simulink model "Waehrungsmodelle"  (R2014a)
settings: Solver=ode1  StartTime=0.0  StopTime=100  FixedStep=1  MaxStep=1  MinStep=1  RelTol=1e-3
(part 8 of 18)

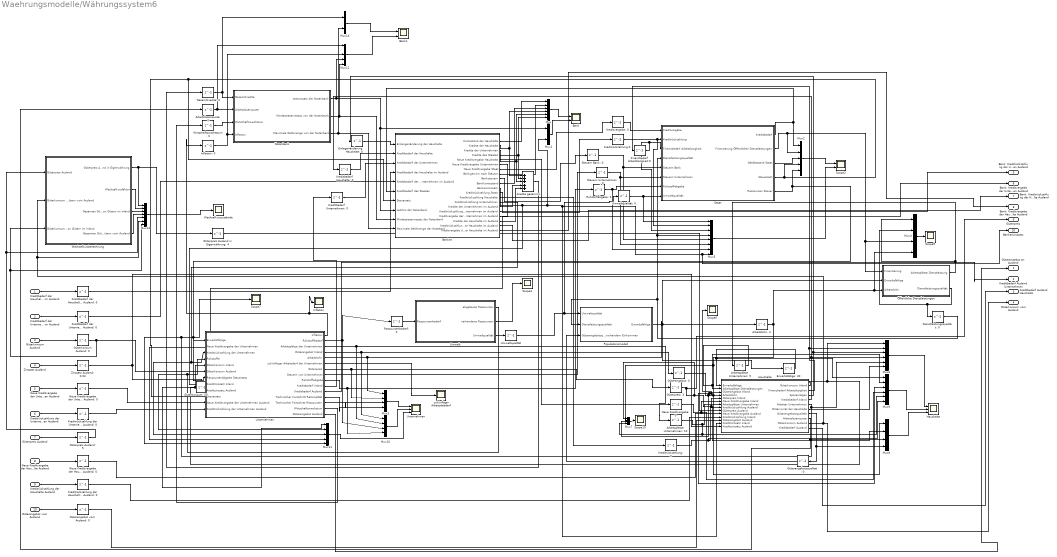
== system Waehrungsmodelle/Währungssystem6 ==
  Kreditbedarf der Haushalte im Ausland : Inport
  Kreditbedarf der Unternehmen im Ausland : Inport  Port=2
  Güterkonsum Ausland : Inport  Port=3
  Zinssatz Ausland : Inport  Port=4
  Neue Kreditvergabe der Unternehmen Ausland : Inport  Port=5
  Kreditrückzahlung der Unternehmen Ausland : Inport  Port=6
  Güterpreis Ausland : Inport  Port=7
  Neue Kreditvergabe der Haushalte Ausland : Inport  Port=8
  Kreditrückzahlung der Haushalte Ausland : Inport  Port=9
  Güterangebot vom  Ausland : Inport  Port=10
  Arbeitslohn: 4 : Delay  DelayLength=1  InitialCondition=4
  Arbeitslosenquote: 0 : Delay  DelayLength=1  InitialCondition=0
  "Arbeitsplätze Unternehmen: 10 " : Delay  DelayLength=1  InitialCondition=10
  Arbeitsplätze Unternehmen: 5 : Delay  DelayLength=1  InitialCondition=5
  Bank : Scope  NumInputPorts=2
      settings: ShowLegends=on  TimeRange=20  YMin=-500~0  YMax=500~0.1
  Bank1 : Scope  NumInputPorts=2
      settings: ShowLegends=on  TimeRange=20  YMin=-500~-0.5  YMax=10000~0.5  SaveName=ScopeData3
  Banken : Subsystem
  Dienstleistungsqualität: 0 : Delay  DelayLength=1  InitialCondition=0
  Einlagenänderung Haushalte: 0 : Delay  DelayLength=1  InitialCondition=0
  Erwerbstätige: 30 : Delay  DelayLength=1  InitialCondition=30
  Finanzbedarf Arbeitslosigkeit:0 : Delay  DelayLength=1  InitialCondition=0
  Gesamtkredite: 0 : Delay  DelayLength=1  InitialCondition=0
  Güterangebot vom  Ausland: 0 : Delay  DelayLength=1  InitialCondition=0
  Güterangebot: 0 : Delay  DelayLength=1  InitialCondition=0
  Güterangebotsqualität: 0 : Delay  DelayLength=1  InitialCondition=0
  Güterkonsum Ausland: 0 : Delay  DelayLength=1  InitialCondition=0
  Güterkonsum: 50 : Delay  DelayLength=1  InitialCondition=50
  Güterpreis Ausland in Eigenwährung: 4 : Delay  DelayLength=1  InitialCondition=4
  Güterpreis Ausland: 5 : Delay  DelayLength=1  InitialCondition=5
  Güterpreis: 3 : Delay  DelayLength=1  InitialCondition=3
  Haushalte : Subsystem
  "Haushalte " : Scope  NumInputPorts=3
      settings: TickLabels=on  ShowLegends=on  TimeRange=100  YMin=-50~0~0  YMax=150~100~1
  Inflation : Scope
      settings: ShowLegends=on  TimeRange=100  YMin=-0.1  YMax=0.15  SaveName=ScopeData12
  Inflation: 0 : Delay  DelayLength=1  InitialCondition=0
  Kreditbedarf Haushalte: 0 : Delay  DelayLength=1  InitialCondition=0
  Kreditbedarf Unternehmen: 0 : Delay  DelayLength=1  InitialCondition=0
  Kreditbedarf der Haushalte im Ausland: 0 : Delay  DelayLength=1  InitialCondition=0
  Kreditbedarf der Unternehmen im Ausland: 0 : Delay  DelayLength=1  InitialCondition=0
  Kredite gesammt : Sum  Inputs=+++++
  Kreditrückzahlung der Haushalte Ausland: 0 : Delay  DelayLength=1  InitialCondition=0
  Kreditrückzahlung der Unternehmen Ausland: 0 : Delay  DelayLength=1  InitialCondition=0
  Kreditrückzahlung: 0 : Delay  DelayLength=1  InitialCondition=0
  Kreditrückzahlung:0 : Delay  DelayLength=1  InitialCondition=0
  Kreditvergabe: 0 : Delay  DelayLength=1  InitialCondition=0
  Mux : Mux  Inputs=6
  Mux1 : Mux  Inputs=2
  Mux{3..4,7..8,10} (5 alike) : Mux
  Mux11 : Mux  Inputs=5
  Mux12 : Mux  Inputs=5
  Mux13 : Mux  Inputs=7
  Mux14 : Mux  Inputs=2
  Mux2 : Mux  Inputs=5
  Mux5 : Mux  Inputs=8
  Mux6 : Mux  Inputs=6
  Mux9 : Mux  Inputs=6
  Neue Kreditvergabe der Haushalte Ausland: 0 : Delay  DelayLength=1  InitialCondition=0
  Neue Kreditvergabe der Unternehmen Ausland: 0 : Delay  DelayLength=1  InitialCondition=0
  Neue Kreditvergabe: 0 : Delay  DelayLength=1  InitialCondition=0
  Notenbank : Subsystem
  Populationsmodell : Subsystem
  Ressourcenbedarf: 0 : Delay  DelayLength=1  InitialCondition=0
  Rohstoffabgabe: 0 : Delay  DelayLength=1  InitialCondition=0
  Scope{4..5,7,9..10} (5 alike) : Scope
      Scope10 settings: ShowLegends=on  TimeRange=100  YMin=0  YMax=120  SaveName=ScopeData10
      Scope4 settings: SaveName=ScopeData4
      Scope5 settings: TimeRange=10  YMin=0  YMax=10  SaveName=ScopeData5
      Scope7 settings: ShowLegends=on  TimeRange=10  YMin=9  YMax=15  SaveName=ScopeData7
      Scope9 settings: TickLabels=on  ShowLegends=on  TimeRange=100  YMin=0  YMax=40  SaveName=ScopeData9
  Scope2 : Scope  NumInputPorts=2
      settings: ShowLegends=on  TimeRange=100  YMin=-100~0  YMax=300~500  SaveName=ScopeData2
  Staat : Subsystem
  Steuern Bank: 0 : Delay  DelayLength=1  InitialCondition=0
  Steuern Unternehmen: 0 : Delay  DelayLength=1  InitialCondition=0
  Umwelt : Subsystem
  Umweltqualität : Delay  DelayLength=1  InitialCondition=0
  Umweltqualität: 0 : Delay  DelayLength=1  InitialCondition=0
  Unternehmen : Subsystem
  "Unternehmen " : Scope  NumInputPorts=3
      settings: TickLabels=on  ShowLegends=on  TimeRange=100  YMin=2~-5~-5  YMax=50~200~100  SaveName=ScopeData6
  Wechselkursberechnung : Subsystem
  Wechselkurszustände : Scope
      settings: ShowLegends=on  TimeRange=100  YMin=0  YMax=1  SaveName=ScopeData11
  Wirtschaftswachtstum: 0 : Delay  DelayLength=1  InitialCondition=0
  Zinssatz Ausland: 0.03 : Delay  DelayLength=1  InitialCondition=0.03
  zukünftiger Arbeitsdebdarf : Scope
      settings: ShowLegends=on  TimeRange=10  YMin=9  YMax=15  SaveName=ScopeData14
  Öffentliche Dienstleistungen : Subsystem
  Güterangebot an  Ausland : Outport
  Kreditbedarf Ausland Unternehmen : Outport  Port=2
  Kreditbedarf Ausland Haushalte : Outport  Port=3
  Güterkonsum vom Ausland : Outport  Port=4
  Bank: Kreditrückzahlung der Unternemen Ausland : Outport  Port=5
  "Bank: Kreditvergabe der Unternemen Ausland " : Outport  Port=6
  Bank: Kreditrückzahlung der Haushalte Ausland : Outport  Port=7
  "Bank: Kreditvergabe der Haushalte Ausland " : Outport  Port=8
  Güterpreis : Outport  Port=9
  Bankenzinssatz : Outport  Port=10
  wires:
  Öffentliche Dienstleistungen/1(Arbeitsplätze Dienstleistung) -> Arbeitsplätze Unternehmen: 5/1, Mux4/1
  Staat/4(Steuersatz) -> Mux2/4, Banken/7(Steuersatz), Unternehmen/10(Steuersatz)
  Umwelt/3(Umweltqualität) -> Umweltqualität/1
  Staat/5(Ressourcen Steuer) -> Unternehmen/7(RessourcenAbgabe Steuersatz), Mux2/5
  Populationsmodell/1(Erwerbsfähige) -> Erwerbstätige: 30/1, Öffentliche Dienstleistungen/2(Erwerbsfähige)
  Unternehmen/7(Güterpreis) -> Mux3/2, Güterpreis: 3/1
  Unternehmen/5(Arbeitslohn) -> Mux3/1, Arbeitslohn: 4/1
  Unternehmen/4(Güterangebot Inland) -> Mux10/1, Güterangebot: 0/1
  Unternehmen/3(Arbeitsplätze der Unternehmen) -> Mux10/2, "Arbeitsplätze Unternehmen: 10 "/1
  Umwelt/1(abgebaute Ressourcen) -> Unternehmen/4(Rohstoffe), Mux11/2
  Haushalte/1(Güterkonsum Inland) -> Mux6/1, Güterkonsum: 50/1
  Haushalte/7(Güterangebotsqualität) -> Mux8/4, Güterangebotsqualität: 0/1
  Staat/2(Finanzierung Öffentlicher Dienstleistungen) -> Mux2/2, Öffentliche Dienstleistungen/1(Finanzierung), Mux4/3
  Haushalte/5(Arbeiter Unternehmen) -> Mux6/5, Scope7/1, Unternehmen/1(Erwerbsfähige), Mux11/5
  Haushalte/2(Finanzbedarf Arbeitslosigkeit) -> Finanzbedarf Arbeitslosigkeit:0/1, Mux6/2
  Unternehmen/8(Steuern von Unternehmen) -> Steuern Unternehmen: 0/1
  Unternehmen/9(Rohstoffabgabe) -> Mux10/4, Rohstoffabgabe: 0/1
  Haushalte/8(Arbeitslosenquote) -> Arbeitslosenquote: 0/1, Mux8/3
  Unternehmen/1(Inflation) -> Inflation/1, Inflation: 0/1
  Unternehmen/14(Wirtschaftswachstum) -> Wirtschaftswachtstum: 0/1
  Notenbank/1(Leitzinssatz der Notenbank) -> Mux12/4, Mux1/1, Banken/8(Leitzins der Notenbank)
  Notenbank/2(Mindestreservesatz von der Notenbank) -> Mux12/5, Banken/9(Mindestreservesatz der Notenbank)
  Notenbank/3(Maximale Geldmenge von der Notenbank) -> Banken/10(Maximale Geldmenge der Notebank), Mux14/2
  Banken/2(Kredite der Haushalte) -> Mux/4, Kredite gesammt/1
  Banken/3(Kredite der Unternehmen) -> Mux/6, Kredite gesammt/2
  Banken/4(Kredite des Staates) -> Mux/5, Kredite gesammt/3
  Banken/9(Banksteuern) -> Steuern Bank: 0/1
  Banken/7(Neue Kreditvergabe Staat) -> Kreditvergabe: 0/1
  Banken/12(Kreditrückzahlung Staat) -> Kreditrückzahlung:0/1
  Banken/13(Kreditrückzahlung Haushalte) -> Kreditrückzahlung: 0/1
  Banken/5(Neue Kreditvergabe Haushalte) -> Neue Kreditvergabe: 0/1
  Haushalte/3(Spareinlagen) -> Einlagenänderung Haushalte: 0/1, Mux6/3
  Haushalte/4(Kreditbedarf Inland) -> Kreditbedarf Haushalte: 0/1, Mux6/4
  Unternehmen/10(Kreditbedarf Inland) -> Kreditbedarf Unternehmen: 0/1
  Staat/1(Kreditbedarf) -> Banken/6(Kreditbedarf des Staates), Mux2/1
  Banken/6(Neue Kreditvergabe Unternehmen) -> Mux11/4, Unternehmen/2(Neue Kreditvergabe der Unternehmen)
  Banken/14(Kreditrückzahlung Unternehmen) -> Unternehmen/3(Kreditrückzahlung der Unternehmen), Mux11/3
  Banken/1(Kontostand der Haushalte) -> Mux/1
  Banken/8(Bankgewinn nach Steuern) -> Mux/2
  Banken/10(Bankkontostand) -> Mux/3
  Banken/11(Bankenzinssatz) -> Haushalte/13(Kreditzinssatz Inland), Bankenzinssatz/1, Mux5/8, Mux1/2, Unternehmen/8(Kreditzinssatz Inland)
  Unternehmen/13(Technischer Fortschritt Ressourcen) -> Mux3/3
  Unternehmen/12(Technischer Fortschritt Rationalität) -> Mux3/4
  Umwelt/2(verhandene Ressourcen) -> Scope4/1
  Kredite gesammt/1 -> Gesamtkredite: 0/1
  Gesamtkredite: 0/1 -> Notenbank/1(Gesamtkredite), Mux14/1
  Wirtschaftswachtstum: 0/1 -> Notenbank/3(Wirtschaftswachtsum)
  Inflation: 0/1 -> Mux12/3, Notenbank/4(Inflation)
  Ressourcenbedarf: 0/1 -> Umwelt/1(Ressourcenbedarf)
  Unternehmen/2(Rohstoffbedarf) -> Ressourcenbedarf: 0/1, Mux10/3
  Umweltqualität: 0/1 -> Mux5/1, Staat/8(Umweltqualität)
  Rohstoffabgabe: 0/1 -> Mux5/7, Staat/7(Rohstoffabgabe)
  Dienstleistungsqualität: 0/1 -> Populationsmodell/2(Dienstleistungsqualität), Staat/4(Dienstleistungsqualität), Mux5/4
  Steuern Unternehmen: 0/1 -> Mux5/6, Staat/6(Steuern Unternehmen)
  Steuern Bank: 0/1 -> Staat/5(Steuern Bank), Mux5/5
  Finanzbedarf Arbeitslosigkeit:0/1 -> Mux5/3, Staat/3(Finanzbedarf Arbeitslosigkeit)
  Kreditrückzahlung:0/1 -> Staat/2(Kreditrückzahlung), Mux5/2
  Kreditvergabe: 0/1 -> Staat/1(Kreditvergabe)
  Umweltqualität/1 -> Umweltqualität: 0/1, Populationsmodell/1(Umweltqualität)
  Öffentliche Dienstleistungen/2(Dienstleistungsqualität) -> Dienstleistungsqualität: 0/1, Mux4/2
  Güterangebotsqualität: 0/1 -> Populationsmodell/3(Güterangebotsqualität bei vorhandem Einkommen)
  "Arbeitsplätze Unternehmen: 10 "/1 -> Mux9/5, Mux7/4, Haushalte/7(Arbeitsplätze Unternehmen)
  Kreditrückzahlung: 0/1 -> Mux9/6, Haushalte/8(Kreditrückzahlung Ausland)
  Neue Kreditvergabe: 0/1 -> Mux9/4, Haushalte/6(Neue Kreditvergabe Inland)
  Arbeitslohn: 4/1 -> Mux8/1, Haushalte/4(Arbeitslohn), Mux7/2, Mux4/4, Öffentliche Dienstleistungen/3(Arbeitslohn)
  Güterangebot: 0/1 -> Mux7/3, Mux9/3, Haushalte/3(Güterangebot Inland), Scope5/1
  Arbeitsplätze Unternehmen: 5/1 -> Haushalte/2(Arbeitsplätze Dienstleistungen), Mux9/2
  Erwerbstätige: 30/1 -> Haushalte/1(Erwerbsfähige), Mux9/1
  Güterkonsum: 50/1 -> Unternehmen/5(Güterkonsum Inland), Mux11/1
  Mux4/1 -> Scope9/1
  Staat/3(Geldbestand Staat) -> Mux2/3
  Mux2/1 -> Scope2/1
  Mux5/1 -> Scope2/2
  Mux/1 -> Bank/1
  Mux7/1 -> Scope10/1
  Mux1/1 -> Bank/2
  Mux6/1 -> "Haushalte "/1
  Mux8/1 -> "Haushalte "/3
  Haushalte/6(Gütervorrat der Haushalte) -> Mux6/6
  Mux9/1 -> "Haushalte "/2
  Mux3/1 -> "Unternehmen "/1
  Mux10/1 -> "Unternehmen "/2
  Mux11/1 -> "Unternehmen "/3
  Güterkonsum Ausland/1 -> Güterkonsum Ausland: 0/1
  Zinssatz Ausland: 0.03/1 -> Haushalte/14(Kreditzinssatz Ausland), Unternehmen/9(Kreditzinssatz Ausland)
  Unternehmen/15(Güterangebot Ausland) -> Güterangebot an  Ausland/1
  Kreditbedarf Haushalte: 0/1 -> Banken/2(Kreditbedarf der Haushalte)
  Kreditbedarf Unternehmen: 0/1 -> Banken/3(Kreditbedarf der Unternehmen)
  Einlagenänderung Haushalte: 0/1 -> Banken/1(Einlangenänderung der Haushalte)
  Kreditbedarf der Haushalte im Ausland: 0/1 -> Banken/4(Kreditbedarf der Haushalte im Ausland)
  Kreditbedarf der Unternehmen im Ausland: 0/1 -> Banken/5(Kreditbedarf der Unternehmen im Ausland)
  Neue Kreditvergabe der Unternehmen Ausland/1 -> Neue Kreditvergabe der Unternehmen Ausland: 0/1
  Kreditrückzahlung der Unternehmen Ausland/1 -> Kreditrückzahlung der Unternehmen Ausland: 0/1
  Banken/16(Kreditrückzahlung der Unternehmen im Ausland) -> Bank: Kreditrückzahlung der Unternemen Ausland/1
  Banken/18(Kredite der Haushalte im Ausland) -> Kredite gesammt/5
  Banken/15(Kredite der Unternehmen im Ausland) -> Kredite gesammt/4
  Neue Kreditvergabe der Haushalte Ausland/1 -> Neue Kreditvergabe der Haushalte Ausland: 0/1
  Unternehmen/11(Kreditbedarf Ausland) -> Kreditbedarf Ausland Unternehmen/1
  Kreditrückzahlung der Haushalte Ausland/1 -> Kreditrückzahlung der Haushalte Ausland: 0/1
  Haushalte/10(Kreditbedarf Ausland) -> Kreditbedarf Ausland Haushalte/1
  Banken/20(Kreditvergabe der Haushalte im Ausland) -> "Bank: Kreditvergabe der Haushalte Ausland "/1
  Güterangebot vom  Ausland/1 -> Güterangebot vom  Ausland: 0/1
  Unternehmen/6(zukünftiger Arbeitsdarf der Unternehmen) -> zukünftiger Arbeitsdebdarf/1
  Banken/17(Kreditvergabe der Unternehmen im Ausland) -> "Bank: Kreditvergabe der Unternemen Ausland "/1
  Banken/19(Kreditrückzahlung der Haushalte im Ausland) -> Bank: Kreditrückzahlung der Haushalte Ausland/1
  Güterpreis: 3/1 -> Güterpreis/1, Mux7/1, Mux8/2, Haushalte/5(Güterpreis Inland)
  Kreditbedarf der Haushalte im Ausland/1 -> Kreditbedarf der Haushalte im Ausland: 0/1
  Kreditbedarf der Unternehmen im Ausland/1 -> Kreditbedarf der Unternehmen im Ausland: 0/1
  Güterkonsum Ausland: 0/1 -> Mux13/7, Wechselkursberechnung/3(Güterkonsum im Ausland von Gütern im Inland), Unternehmen/6(Güterkonsum Ausland)
  Zinssatz Ausland/1 -> Zinssatz Ausland: 0.03/1
  Neue Kreditvergabe der Unternehmen Ausland: 0/1 -> Unternehmen/11(Neue Kreditvergabe der Unternehmen Ausland)
  Kreditrückzahlung der Unternehmen Ausland: 0/1 -> Unternehmen/12(Kreditrückzahlung der Unternehmen Ausland)
  Güterpreis Ausland: 5/1 -> Mux13/5, Wechselkursberechnung/1(Güterpreis Ausland)
  Neue Kreditvergabe der Haushalte Ausland: 0/1 -> Haushalte/10(Neue Kreditvergabe Ausland)
  Kreditrückzahlung der Haushalte Ausland: 0/1 -> Haushalte/11(Kreditrückzahlung Inland)
  Güterangebot vom  Ausland: 0/1 -> Haushalte/12(Güterangebot Ausland)
  Mux14/1 -> Bank1/1
  Mux12/1 -> Bank1/2
  Arbeitslosenquote: 0/1 -> Notenbank/2(Arbeitslosenquote), Mux12/1
  Güterpreis Ausland/1 -> Güterpreis Ausland: 5/1
  Wechselkursberechnung/1(Güterpreis Ausland in Eigenwährung) -> Güterpreis Ausland in Eigenwährung: 4/1, Mux13/1
  Haushalte/9(Güterkonsum Ausland) -> Mux13/6, Wechselkursberechnung/2(Güterkonsum im Inland von Gütern vom Ausland), Güterkonsum vom Ausland/1
  Güterpreis Ausland in Eigenwährung: 4/1 -> Haushalte/9(Güterpreis Ausland)
  Wechselkursberechnung/3(Gesamter Güterkonsum im Ausland von Gütern im Inland) -> Mux13/3
  Wechselkursberechnung/2(Wechselkursfaktor) -> Mux13/2
  Wechselkursberechnung/4(Gesamter Güterkonsum im Inland von Gütern vom Ausland) -> Mux13/4
  Mux13/1 -> Wechselkurszustände/1

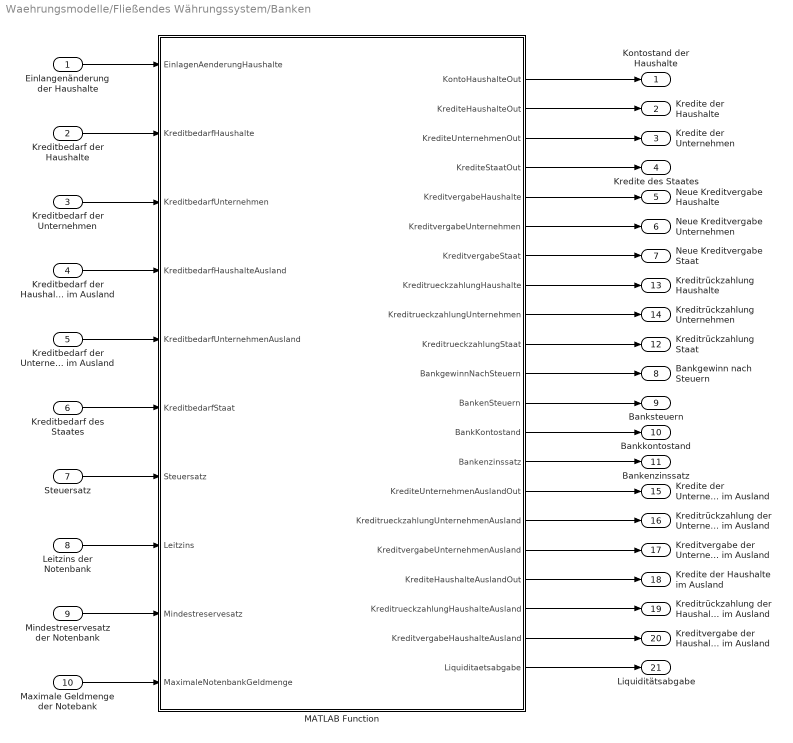
== system Waehrungsmodelle/Fließendes Währungssystem/Banken ==
  Einlangenänderung der Haushalte : Inport
  Kreditbedarf der Haushalte : Inport  Port=2
  Kreditbedarf der Unternehmen : Inport  Port=3
  Kreditbedarf der Haushalte im Ausland : Inport  Port=4
  Kreditbedarf der Unternehmen im Ausland : Inport  Port=5
  Kreditbedarf des Staates : Inport  Port=6
  Steuersatz : Inport  Port=7
  Leitzins der Notenbank : Inport  Port=8
  Mindestreservesatz der Notenbank : Inport  Port=9
  Maximale Geldmenge der Notebank : Inport  Port=10
  MATLAB Function : MATLAB Function  TreatAsAtomicUnit=on
  Kontostand der Haushalte : Outport
  Kredite der Haushalte : Outport  Port=2
  Kredite der Unternehmen : Outport  Port=3
  Kredite des Staates : Outport  Port=4
  Neue Kreditvergabe Haushalte : Outport  Port=5
  Neue Kreditvergabe Unternehmen : Outport  Port=6
  Neue Kreditvergabe Staat : Outport  Port=7
  Bankgewinn nach Steuern : Outport  Port=8
  Banksteuern : Outport  Port=9
  Bankkontostand : Outport  Port=10
  Bankenzinssatz : Outport  Port=11
  Kreditrückzahlung Staat : Outport  Port=12
  Kreditrückzahlung Haushalte : Outport  Port=13
  Kreditrückzahlung Unternehmen : Outport  Port=14
  Kredite der Unternehmen im Ausland : Outport  Port=15
  Kreditrückzahlung der Unternehmen im Ausland : Outport  Port=16
  Kreditvergabe der Unternehmen im Ausland : Outport  Port=17
  Kredite der Haushalte im Ausland : Outport  Port=18
  Kreditrückzahlung der Haushalte im Ausland : Outport  Port=19
  Kreditvergabe der Haushalte im Ausland : Outport  Port=20
  Liquiditätsabgabe : Outport  Port=21
  wires:
  MATLAB Function/1(KontoHaushalteOut) -> Kontostand der Haushalte/1
  MATLAB Function/2(KrediteHaushalteOut) -> Kredite der Haushalte/1
  MATLAB Function/3(KrediteUnternehmenOut) -> Kredite der Unternehmen/1
  MATLAB Function/4(KrediteStaatOut) -> Kredite des Staates/1
  MATLAB Function/5(KreditvergabeHaushalte) -> Neue Kreditvergabe Haushalte/1
  MATLAB Function/6(KreditvergabeUnternehmen) -> Neue Kreditvergabe Unternehmen/1
  MATLAB Function/7(KreditvergabeStaat) -> Neue Kreditvergabe Staat/1
  MATLAB Function/11(BankgewinnNachSteuern) -> Bankgewinn nach Steuern/1
  MATLAB Function/10(KreditrueckzahlungStaat) -> Kreditrückzahlung Staat/1
  MATLAB Function/9(KreditrueckzahlungUnternehmen) -> Kreditrückzahlung Unternehmen/1
  MATLAB Function/8(KreditrueckzahlungHaushalte) -> Kreditrückzahlung Haushalte/1
  MATLAB Function/14(Bankenzinssatz) -> Bankenzinssatz/1
  MATLAB Function/13(BankKontostand) -> Bankkontostand/1
  MATLAB Function/12(BankenSteuern) -> Banksteuern/1
  MATLAB Function/15(KrediteUnternehmenAuslandOut) -> Kredite der Unternehmen im Ausland/1
  MATLAB Function/16(KreditrueckzahlungUnternehmenAusland) -> Kreditrückzahlung der Unternehmen im Ausland/1
  MATLAB Function/17(KreditvergabeUnternehmenAusland) -> Kreditvergabe der Unternehmen im Ausland/1
  MATLAB Function/18(KrediteHaushalteAuslandOut) -> Kredite der Haushalte im Ausland/1
  MATLAB Function/20(KreditvergabeHaushalteAusland) -> Kreditvergabe der Haushalte im Ausland/1
  MATLAB Function/19(KreditrueckzahlungHaushalteAusland) -> Kreditrückzahlung der Haushalte im Ausland/1
  Einlangenänderung der Haushalte/1 -> MATLAB Function/1(EinlagenAenderungHaushalte)
  Kreditbedarf der Haushalte/1 -> MATLAB Function/2(KreditbedarfHaushalte)
  Kreditbedarf der Unternehmen/1 -> MATLAB Function/3(KreditbedarfUnternehmen)
  Kreditbedarf der Haushalte im Ausland/1 -> MATLAB Function/4(KreditbedarfHaushalteAusland)
  Kreditbedarf der Unternehmen im Ausland/1 -> MATLAB Function/5(KreditbedarfUnternehmenAusland)
  Kreditbedarf des Staates/1 -> MATLAB Function/6(KreditbedarfStaat)
  Steuersatz/1 -> MATLAB Function/7(Steuersatz)
  Leitzins der Notenbank/1 -> MATLAB Function/8(Leitzins)
  Mindestreservesatz der Notenbank/1 -> MATLAB Function/9(Mindestreservesatz)
  Maximale Geldmenge der Notebank/1 -> MATLAB Function/10(MaximaleNotenbankGeldmenge)
  MATLAB Function/21(Liquiditaetsabgabe) -> Liquiditätsabgabe/1

== system Waehrungsmodelle/Fließendes Währungssystem/Haushalte ==
  Erwerbsfähige : Inport
  Arbeitsplätze Dienstleistungen : Inport  Port=2
  Güterangebot Inland : Inport  Port=3
  Arbeitslohn : Inport  Port=4
  Güterpreis Inland : Inport  Port=5
  Neue Kreditvergabe Inland : Inport  Port=6
  Arbeitsplätze Unternehmen : Inport  Port=7
  Kreditrückzahlung Ausland : Inport  Port=8
  Güterpreis Ausland : Inport  Port=9
  Neue Kreditvergabe Ausland : Inport  Port=10
  Kreditrückzahlung Inland : Inport  Port=11
  Güterangebot Ausland : Inport  Port=12
  Kreditzinssatz Inland : Inport  Port=13
  Kreditzinssatz Ausland : Inport  Port=14
  MATLAB Function : MATLAB Function  TreatAsAtomicUnit=on
  Güterkonsum Inland : Outport
  Finanzbedarf Arbeitslosigkeit : Outport  Port=2
  Spareinlagen : Outport  Port=3
  Kreditbedarf Inland : Outport  Port=4
  Arbeiter Unternehmen : Outport  Port=5
  Gütervorrat der Haushalte : Outport  Port=6
  Güterangebotsqualität : Outport  Port=7
  Arbeitslosenquote : Outport  Port=8
  Güterkonsum Ausland : Outport  Port=9
  Kreditbedarf Ausland : Outport  Port=10
  wires:
  Arbeitslohn/1 -> MATLAB Function/7(Arbeitslohn)
  Erwerbsfähige/1 -> MATLAB Function/1(Erwerbsfaehige)
  Arbeitsplätze Dienstleistungen/1 -> MATLAB Function/2(ArbeitsplaetzeDienstleistungen)
  Güterangebot Inland/1 -> MATLAB Function/6(GueterAngebotInland)
  Güterpreis Inland/1 -> MATLAB Function/8(GueterpreisInland)
  MATLAB Function/1(GueterkonsumInland) -> Güterkonsum Inland/1
  MATLAB Function/2(FinanzierungArbeitslosigkeit) -> Finanzbedarf Arbeitslosigkeit/1
  MATLAB Function/4(KreditbedarfInland) -> Kreditbedarf Inland/1
  MATLAB Function/5(ArbeiterUnternehmen) -> Arbeiter Unternehmen/1
  MATLAB Function/3(Spareinlagen) -> Spareinlagen/1
  Neue Kreditvergabe Inland/1 -> MATLAB Function/4(NeueKreditvergabeInland)
  Arbeitsplätze Unternehmen/1 -> MATLAB Function/3(ArbeitsplaetzeUnternehmen)
  MATLAB Function/6(GueterVorratHaushalte) -> Gütervorrat der Haushalte/1
  MATLAB Function/7(GueterangebotsqualitaetOut) -> Güterangebotsqualität/1
  Kreditrückzahlung Ausland/1 -> MATLAB Function/5(KreditrueckzahlungInland)
  MATLAB Function/8(Arbeitslosenquote) -> Arbeitslosenquote/1
  MATLAB Function/9(GueterkonsumAusland) -> Güterkonsum Ausland/1
  MATLAB Function/10(KreditbedarfAusland) -> Kreditbedarf Ausland/1
  Güterpreis Ausland/1 -> MATLAB Function/9(GueterpreisAusland)
  Neue Kreditvergabe Ausland/1 -> MATLAB Function/10(NeueKreditvergabeAusland)
  Kreditrückzahlung Inland/1 -> MATLAB Function/11(KreditrueckzahlungAusland)
  Güterangebot Ausland/1 -> MATLAB Function/12(GueterAngebotAusland)
  Kreditzinssatz Inland/1 -> MATLAB Function/13(KreditZinssatzInland)
  Kreditzinssatz Ausland/1 -> MATLAB Function/14(KreditZinssatzAusland)

== system Waehrungsmodelle/Fließendes Währungssystem/Notenbank ==
  Gesamtkredite : Inport
  Arbeitslosenquote : Inport  Port=2
  Wirtschaftswachtsum : Inport  Port=3
  Inflation : Inport  Port=4
  MATLAB Function : MATLAB Function  TreatAsAtomicUnit=on
  Leitzinssatz der Notenbank : Outport
  Mindestreservesatz von der Notenbank : Outport  Port=2
  Maximale Geldmenge von der Notenbank : Outport  Port=3
  wires:
  MATLAB Function/2(MindestreservesatzOut) -> Mindestreservesatz von der Notenbank/1
  MATLAB Function/3(MaximaleNotenbankGeldmengeOut) -> Maximale Geldmenge von der Notenbank/1
  MATLAB Function/1(LeitzinsOut) -> Leitzinssatz der Notenbank/1
  Wirtschaftswachtsum/1 -> MATLAB Function/4(Wirtschaftswachtsum)
  Arbeitslosenquote/1 -> MATLAB Function/2(Arbeitslosenquote)
  Gesamtkredite/1 -> MATLAB Function/1(Gesamtkredite)
  Inflation/1 -> MATLAB Function/3(Inflation)

== system Waehrungsmodelle/Fließendes Währungssystem/Populationsmodell ==
  note: Geburten
  Umweltqualität : Inport
  Dienstleistungsqualität : Inport  Port=2
  Güterangebotsqualität bei vorhandem Einkommen : Inport  Port=3
  Ausgleichsfaktor : Constant  Value=0.3
  Dienstleistungs- multiplikator : Sum
  Divide1 : Product  Inputs=*/
  Divide2 : Product  Inputs=*/
  Divide3 : Product  Inputs=*/
  Erwachsene : Sum  Inputs=+--
  Fertilitätsmultiplikator : Product  Inputs=4
  Fertilitätsrate pro Frau : Constant  Value=3/40
  Frauenanteil pro Erwachsene : Constant  Value=0.5
  Güterangebotsqualitäts- multiplikator : Sum
  Jahre der Altersklasse : Constant  Value=15
  Jahre der Altersklasse1 : Constant  Value=10
  Jahre der Altersklasse2 : Constant  Value=40
  Kinder : Sum  Inputs=+--
  Lebensqualitätsfaktor : Product  Inputs=/
  Product{,1..3} (4 alike) : Product  Inputs=3
  Schüler / Studenten : Sum  Inputs=+--
  Start Erwachsene: 55 : Integrator  InitialCondition=55
  Start Kinder: 13 : Integrator  InitialCondition=13
  Start Schüler: 11 : Integrator  InitialCondition=11
  Sterblichkeitsrate Kinder : Constant  Value=0.003
  Sterblichkeitsrate1 : Constant  Value=0.002
  Sterblichkeitsrate2 : Constant  Value=0.004
  Umwelt- multiplikator : Sum
  Erwerbsfähige : Outport
  wires:
  Product/1 -> Kinder/1
  Jahre der Altersklasse2/1 -> Divide3/2
  Jahre der Altersklasse/1 -> Divide1/2
  Divide1/1 -> Schüler / Studenten/1, Kinder/3
  Sterblichkeitsrate1/1 -> Product1/2
  Sterblichkeitsrate Kinder/1 -> Product2/2
  Divide2/1 -> Schüler / Studenten/3, Erwachsene/1
  Start Schüler: 11/1 -> Product1/3, Divide2/1
  Jahre der Altersklasse1/1 -> Divide2/2
  Sterblichkeitsrate2/1 -> Product3/2
  Start Erwachsene: 55/1 -> Erwerbsfähige/1, Product3/3, Divide3/1, Product/1
  Erwachsene/1 -> Start Erwachsene: 55/1
  Kinder/1 -> Start Kinder: 13/1
  Start Kinder: 13/1 -> Product2/3, Divide1/1
  Schüler / Studenten/1 -> Start Schüler: 11/1
  Ausgleichsfaktor/1 -> Umwelt- multiplikator/2, Güterangebotsqualitäts- multiplikator/1, Dienstleistungs- multiplikator/1
  Fertilitätsmultiplikator/1 -> Product/3
  Umweltqualität/1 -> Umwelt- multiplikator/1
  Dienstleistungs- multiplikator/1 -> Lebensqualitätsfaktor/1, Fertilitätsmultiplikator/4
  Fertilitätsrate pro Frau/1 -> Fertilitätsmultiplikator/1
  Umwelt- multiplikator/1 -> Fertilitätsmultiplikator/2
  Dienstleistungsqualität/1 -> Dienstleistungs- multiplikator/2
  Product2/1 -> Kinder/2
  Product1/1 -> Schüler / Studenten/2
  Divide3/1 -> Erwachsene/3
  Product3/1 -> Erwachsene/2
  Lebensqualitätsfaktor/1 -> Product3/1, Product1/1, Product2/1
  Güterangebotsqualität bei vorhandem Einkommen/1 -> Güterangebotsqualitäts- multiplikator/2
  Güterangebotsqualitäts- multiplikator/1 -> Fertilitätsmultiplikator/3
  Frauenanteil pro Erwachsene/1 -> Product/2

== system Waehrungsmodelle/Fließendes Währungssystem/Staat ==
  Kreditvergabe : Inport
  Kreditrückzahlung : Inport  Port=2
  Finanzbedarf Arbeitslosigkeit : Inport  Port=3
  Dienstleistungsqualität : Inport  Port=4
  Steuern Bank : Inport  Port=5
  Steuern Unternehmen : Inport  Port=6
  Rohstoffabgabe : Inport  Port=7
  Umweltqualität : Inport  Port=8
  Liquiditätsabgabe : Inport  Port=9
  MATLAB Function : MATLAB Function  TreatAsAtomicUnit=on
  Kreditbedarf : Outport
  Finanzierung Öffentlicher Dienstleistungen : Outport  Port=2
  Geldbestand Staat : Outport  Port=3
  Steuersatz : Outport  Port=4
  Ressourcen Steuer : Outport  Port=5
  wires:
  Steuern Unternehmen/1 -> MATLAB Function/6(SteuernUnternehmen)
  Dienstleistungsqualität/1 -> MATLAB Function/4(Dienstleistungsqualitaet)
  MATLAB Function/4(SteuersatzOut) -> Steuersatz/1
  MATLAB Function/2(FinanzierungOeffentlicheDienstleistungen) -> Finanzierung Öffentlicher Dienstleistungen/1
  Finanzbedarf Arbeitslosigkeit/1 -> MATLAB Function/3(FinanzbedarfArbeitslosigkeit)
  MATLAB Function/3(GeldbestandStaat) -> Geldbestand Staat/1
  Kreditrückzahlung/1 -> MATLAB Function/2(Kreditrueckzahlung)
  MATLAB Function/1(Kreditbedarf) -> Kreditbedarf/1
  Steuern Bank/1 -> MATLAB Function/5(SteuernBanken)
  Kreditvergabe/1 -> MATLAB Function/1(KreditvergabeNeuStaat)
  MATLAB Function/5(RessourcenAbgabesatzOut) -> Ressourcen Steuer/1
  Rohstoffabgabe/1 -> MATLAB Function/7(Rohstoffabgabe)
  Umweltqualität/1 -> MATLAB Function/8(Umweltqualitaet)
  Liquiditätsabgabe/1 -> MATLAB Function/9(Liquiditaetsabgabe)

== system Waehrungsmodelle/Fließendes Währungssystem/Umwelt ==
  Ressourcenbedarf : Inport
  Umwelt : MATLAB Function  TreatAsAtomicUnit=on
  abgebaute Ressourcen : Outport
  verhandene Ressourcen : Outport  Port=2
  Umweltqualität : Outport  Port=3
  wires:
  Umwelt/3(Umweltqualitaet) -> Umweltqualität/1
  Umwelt/2(VorhandeneRessourcenOut) -> verhandene Ressourcen/1
  Umwelt/1(AbgebauteRessourcen) -> abgebaute Ressourcen/1
  Ressourcenbedarf/1 -> Umwelt/1(Ressourcenbedarf)

== system Waehrungsmodelle/Fließendes Währungssystem/Unternehmen ==
  Erwerbsfähige : Inport
  Neue Kreditvergabe der Unternehmen : Inport  Port=2
  Kreditrückzahlung der Unternehmen : Inport  Port=3
  Rohstoffe : Inport  Port=4
  Güterkonsum Inland : Inport  Port=5
  Güterkonsum Ausland : Inport  Port=6
  RessourcenAbgabe Steuersatz : Inport  Port=7
  Kreditzinssatz Inland : Inport  Port=8
  Kreditzinssatz Ausland : Inport  Port=9
  Steuersatz : Inport  Port=10
  Neue Kreditvergabe der Unternehmen Ausland : Inport  Port=11
  Kreditrückzahlung der Unternehmen Ausland : Inport  Port=12
  MATLAB Function : MATLAB Function  TreatAsAtomicUnit=on
  Inflation : Outport
  Rohstoffbedarf : Outport  Port=2
  Arbeitsplätze der Unternehmen : Outport  Port=3
  Güterangebot Inland : Outport  Port=4
  Arbeitslohn : Outport  Port=5
  zukünftiger Arbeitsdarf der Unternehmen : Outport  Port=6
  Güterpreis : Outport  Port=7
  Steuern von Unternehmen : Outport  Port=8
  Rohstoffabgabe : Outport  Port=9
  Kreditbedarf Inland : Outport  Port=10
  Kreditbedarf Ausland : Outport  Port=11
  Technischer Fortschritt Rationalität : Outport  Port=12
  Technischer Fortschritt Ressourcen : Outport  Port=13
  Wirtschaftswachstum : Outport  Port=14
  Güterangebot Ausland : Outport  Port=15
  wires:
  MATLAB Function/8(SteuernUnternehmen) -> Steuern von Unternehmen/1
  MATLAB Function/7(GueterpreisOut) -> Güterpreis/1
  Neue Kreditvergabe der Unternehmen/1 -> MATLAB Function/2(NeueKreditvergabeUnternehmen)
  Kreditrückzahlung der Unternehmen/1 -> MATLAB Function/3(KreditrueckzahlungUnternehmen)
  MATLAB Function/6(BenoetigterArbeitsbedarfUnternehmen) -> zukünftiger Arbeitsdarf der Unternehmen/1
  MATLAB Function/4(GueterangebotInland) -> Güterangebot Inland/1
  MATLAB Function/5(ArbeitslohnOut) -> Arbeitslohn/1
  MATLAB Function/2(Rohstoffbedarf) -> Rohstoffbedarf/1
  MATLAB Function/1(Inflation) -> Inflation/1
  Erwerbsfähige/1 -> MATLAB Function/1(Erwerbsfaehige)
  MATLAB Function/3(ArbeitsplaetzeUnternehmen) -> Arbeitsplätze der Unternehmen/1
  Rohstoffe/1 -> MATLAB Function/4(Rohstoffe)
  Güterkonsum Inland/1 -> MATLAB Function/5(GueterkonsumInland)
  MATLAB Function/9(RessourcenAbgabeSteuer) -> Rohstoffabgabe/1
  MATLAB Function/11(KreditbedarfAusland) -> Kreditbedarf Ausland/1
  MATLAB Function/12(TechnischeVerbesserungRationalitaetOut) -> Technischer Fortschritt Rationalität/1
  MATLAB Function/13(TechnischeVerbesserungRessourcenOut) -> Technischer Fortschritt Ressourcen/1
  Güterkonsum Ausland/1 -> MATLAB Function/6(GueterkonsumAusland)
  RessourcenAbgabe Steuersatz/1 -> MATLAB Function/7(RessourcenAbgabeSteuersatz)
  Kreditzinssatz Inland/1 -> MATLAB Function/8(KreditZinssatzInland)
  Kreditzinssatz Ausland/1 -> MATLAB Function/9(KreditZinssatzAusland)
  Steuersatz/1 -> MATLAB Function/10(Steuersatz)
  MATLAB Function/10(KreditbedarfInland) -> Kreditbedarf Inland/1
  MATLAB Function/14(Wirtschaftswachstum) -> Wirtschaftswachstum/1
  MATLAB Function/15(GueterangebotAusland) -> Güterangebot Ausland/1
  Neue Kreditvergabe der Unternehmen Ausland/1 -> MATLAB Function/11(NeueKreditvergabeUnternehmenAusland)
  Kreditrückzahlung der Unternehmen Ausland/1 -> MATLAB Function/12(KreditrueckzahlungUnternehmenAusland)

== system Waehrungsmodelle/Fließendes Währungssystem/Wechselkursberechnung ==
  Güterpreis Ausland : Inport
  Güterkonsum im Inland von Gütern vom Ausland : Inport  Port=2
  Güterkonsum im Ausland von Gütern im Inland : Inport  Port=3
  MATLAB Function : MATLAB Function  TreatAsAtomicUnit=on
  Güterpreis Ausland in Eigenwährung : Outport
  Wechselkursfaktor : Outport  Port=2
  Gesamter Güterkonsum im Ausland von Gütern im Inland : Outport  Port=3
  Gesamter Güterkonsum im Inland von Gütern vom Ausland : Outport  Port=4
  wires:
  Güterpreis Ausland/1 -> MATLAB Function/1(GueterpreisAusland)
  Güterkonsum im Inland von Gütern vom Ausland/1 -> MATLAB Function/2(GueterKonsumImInlandVomAusland)
  Güterkonsum im Ausland von Gütern im Inland/1 -> MATLAB Function/3(GueterKonsumImAuslandVomInland)
  MATLAB Function/1(GueterpreisAuslandInEigenwaehrung) -> Güterpreis Ausland in Eigenwährung/1
  MATLAB Function/2(Wechselkursfaktor) -> Wechselkursfaktor/1
  MATLAB Function/3(GesamterGueterKonsumImAuslandVomInlandOut) -> Gesamter Güterkonsum im Ausland von Gütern im Inland/1
  MATLAB Function/4(GesamterGueterKonsumImInlandVomAuslandOut) -> Gesamter Güterkonsum im Inland von Gütern vom Ausland/1

== system Waehrungsmodelle/Fließendes Währungssystem/Öffentliche Dienstleistungen ==
  Finanzierung : Inport
  Erwerbsfähige : Inport  Port=2
  Arbeitslohn : Inport  Port=3
  MATLAB Function : MATLAB Function  TreatAsAtomicUnit=on
  Arbeitsplätze Dienstleistung : Outport
  Dienstleistungsqualität : Outport  Port=2
  wires:
  Arbeitslohn/1 -> MATLAB Function/3(Arbeitslohn)
  Erwerbsfähige/1 -> MATLAB Function/2(Erwerbsfaehige)
  Finanzierung/1 -> MATLAB Function/1(Finanzierung)
  MATLAB Function/1(ArbeitsplaetzeDienstleistung) -> Arbeitsplätze Dienstleistung/1
  MATLAB Function/2(Dienstleistungsqualitaet) -> Dienstleistungsqualität/1

== system Waehrungsmodelle/Freies Geld Währungssystem/Banken ==
  Einlangenänderung der Haushalte : Inport
  Kreditbedarf der Haushalte : Inport  Port=2
  Kreditbedarf der Unternehmen : Inport  Port=3
  Kreditbedarf der Haushalte im Ausland : Inport  Port=4
  Kreditbedarf der Unternehmen im Ausland : Inport  Port=5
  Kreditbedarf des Staates : Inport  Port=6
  Steuersatz : Inport  Port=7
  PreisDeckungsmaterial : Inport  Port=8
  MengeDeckungsmaterial : Inport  Port=9
  MATLAB Function : MATLAB Function  TreatAsAtomicUnit=on
  Kontostand der Haushalte : Outport
  Kredite der Haushalte : Outport  Port=2
  Kredite der Unternehmen : Outport  Port=3
  Kredite des Staates : Outport  Port=4
  Neue Kreditvergabe Haushalte : Outport  Port=5
  Neue Kreditvergabe Unternehmen : Outport  Port=6
  Neue Kreditvergabe Staat : Outport  Port=7
  Bankgewinn nach Steuern : Outport  Port=8
  Banksteuern : Outport  Port=9
  Bankkontostand : Outport  Port=10
  Bankenzinssatz : Outport  Port=11
  Kreditrückzahlung Staat : Outport  Port=12
  Kreditrückzahlung Haushalte : Outport  Port=13
  Kreditrückzahlung Unternehmen : Outport  Port=14
  Kredite der Unternehmen im Ausland : Outport  Port=15
  Kreditrückzahlung der Unternehmen im Ausland : Outport  Port=16
  Kreditvergabe der Unternehmen im Ausland : Outport  Port=17
  Kredite der Haushalte im Ausland : Outport  Port=18
  Kreditrückzahlung der Haushalte im Ausland : Outport  Port=19
  Kreditvergabe der Haushalte im Ausland : Outport  Port=20
  NachfrageDeckungsmaterial : Outport  Port=21
  Maximale Kreditvergabe : Outport  Port=22
  wires:
  Einlangenänderung der Haushalte/1 -> MATLAB Function/1(EinlagenAenderungHaushalte)
  Kreditbedarf der Haushalte/1 -> MATLAB Function/2(KreditbedarfHaushalte)
  Kreditbedarf der Unternehmen/1 -> MATLAB Function/3(KreditbedarfUnternehmen)
  Kreditbedarf der Haushalte im Ausland/1 -> MATLAB Function/4(KreditbedarfHaushalteAusland)
  Kreditbedarf der Unternehmen im Ausland/1 -> MATLAB Function/5(KreditbedarfUnternehmenAusland)
  Kreditbedarf des Staates/1 -> MATLAB Function/6(KreditbedarfStaat)
  Steuersatz/1 -> MATLAB Function/7(Steuersatz)
  MengeDeckungsmaterial/1 -> MATLAB Function/9(MengeDeckungsmaterial)
  PreisDeckungsmaterial/1 -> MATLAB Function/8(PreisDeckungsmaterial)
  MATLAB Function/1(KontoHaushalteOut) -> Kontostand der Haushalte/1
  MATLAB Function/2(KrediteHaushalteOut) -> Kredite der Haushalte/1
  MATLAB Function/3(KrediteUnternehmenOut) -> Kredite der Unternehmen/1
  MATLAB Function/4(KrediteStaatOut) -> Kredite des Staates/1
  MATLAB Function/5(KreditvergabeHaushalte) -> Neue Kreditvergabe Haushalte/1
  MATLAB Function/6(KreditvergabeUnternehmen) -> Neue Kreditvergabe Unternehmen/1
  MATLAB Function/7(KreditvergabeStaat) -> Neue Kreditvergabe Staat/1
  MATLAB Function/8(KreditrueckzahlungHaushalte) -> Kreditrückzahlung Haushalte/1
  MATLAB Function/9(KreditrueckzahlungUnternehmen) -> Kreditrückzahlung Unternehmen/1
  MATLAB Function/10(KreditrueckzahlungStaat) -> Kreditrückzahlung Staat/1
  MATLAB Function/11(BankgewinnNachSteuern) -> Bankgewinn nach Steuern/1
  MATLAB Function/12(BankenSteuern) -> Banksteuern/1
  MATLAB Function/13(BankKontostand) -> Bankkontostand/1
  MATLAB Function/14(Bankenzinssatz) -> Bankenzinssatz/1
  MATLAB Function/15(KrediteUnternehmenAuslandOut) -> Kredite der Unternehmen im Ausland/1
  MATLAB Function/16(KreditrueckzahlungUnternehmenAusland) -> Kreditrückzahlung der Unternehmen im Ausland/1
  MATLAB Function/17(KreditvergabeUnternehmenAusland) -> Kreditvergabe der Unternehmen im Ausland/1
  MATLAB Function/18(KrediteHaushalteAuslandOut) -> Kredite der Haushalte im Ausland/1
  MATLAB Function/19(KreditrueckzahlungHaushalteAusland) -> Kreditrückzahlung der Haushalte im Ausland/1
  MATLAB Function/20(KreditvergabeHaushalteAusland) -> Kreditvergabe der Haushalte im Ausland/1
  MATLAB Function/21(NachfrageDeckungsmaterial) -> NachfrageDeckungsmaterial/1
  MATLAB Function/22(MaximaleKreditvergabe) -> Maximale Kreditvergabe/1

== matlab function Waehrungsmodelle/Freies Geld Währungssystem/Banken/MATLAB Function ==
  data: EinlagenAenderungHaushalte input; KreditbedarfHaushalte input; KreditbedarfUnternehmen input; KreditbedarfHaushalteAusland input; KreditbedarfUnternehmenAusland input; KreditbedarfStaat input; Steuersatz input; PreisDeckungsmaterial input; MengeDeckungsmaterial input; KontoHaushalteOut output; KrediteHaushalteOut output; KrediteUnternehmenOut output; KrediteStaatOut output; KreditvergabeHaushalte output; KreditvergabeUnternehmen output; KreditvergabeStaat output; KreditrueckzahlungHaushalte output; KreditrueckzahlungUnternehmen output; KreditrueckzahlungStaat output; BankgewinnNachSteuern output; BankenSteuern output; BankKontostand output; Bankenzinssatz output; KrediteUnternehmenAuslandOut output; KreditrueckzahlungUnternehmenAusland output; KreditvergabeUnternehmenAusland output; KrediteHaushalteAuslandOut output; KreditrueckzahlungHaushalteAusland output; KreditvergabeHaushalteAusland output; NachfrageDeckungsmaterial output; MaximaleKreditvergabe output
function [KontoHaushalteOut, KrediteHaushalteOut, KrediteUnternehmenOut, KrediteStaatOut, ... 
            KreditvergabeHaushalte, KreditvergabeUnternehmen, KreditvergabeStaat, ...
            KreditrueckzahlungHaushalte, KreditrueckzahlungUnternehmen, KreditrueckzahlungStaat, ...
            BankgewinnNachSteuern, BankenSteuern, BankKontostand, Bankenzinssatz, ...
            KrediteUnternehmenAuslandOut, KreditrueckzahlungUnternehmenAusland, KreditvergabeUnternehmenAusland, ...
            KrediteHaushalteAuslandOut, KreditrueckzahlungHaushalteAusland, KreditvergabeHaushalteAusland, ...
            NachfrageDeckungsmaterial, MaximaleKreditvergabe] = ...
    Banken(EinlagenAenderungHaushalte, KreditbedarfHaushalte, KreditbedarfUnternehmen, ...
            KreditbedarfHaushalteAusland, KreditbedarfUnternehmenAusland, KreditbedarfStaat, ...
            Steuersatz, PreisDeckungsmaterial, MengeDeckungsmaterial)
% Submodell Banken zur Berechnung der Geld-Prozesse zwischen 
% Banken und Haushalten

% ANMERKUNG:
% Warum gibt es auf der einen Seite Kredite und Guthaben der Haushalte?
% Der überwigende Teil der Geldes MUSS den Haushalten gehören, da diese
% die Unternehmen und Banken besitzen. Ich vermute, dass es in einen
% demokratischen Staat nicht möglich ist, dass der Staat mehr Geld als 
% die Bevölkerung besitzt.
% Die ungleiche Geldverteilung ist dafür verantwortlich, dass die Haushalte
% auf der einen Seite Spareinlagen und Kredite haben. Ohne Spareinlagen wäre
% es aktuell nicht möglich Kredite überhaupt zu vergeben.

% Der Zinsspread ist die Prozentuale-Differenz der Zinsweitergabe bei
% Krediten und Anlagen
persistent Zinsspread;

% interner Zinssatz
persistent InternerZinssatz;

% aktuelle Kredithöhe der Unternehmen
persistent KrediteUnternehmen;

% aktuelle Kredithöhe des Staats
persistent KrediteStaat;

% aktuelle Kredithöhe der Haushalte
persistent KrediteHaushalte;

% aktuelle Kredithöhe der Unternehmen im Ausland
persistent KrediteUnternehmenAusland;

% aktuelle Kredithöhe der Haushalte im Ausland
persistent KrediteHaushalteAusland;

% aktueller Kontostand der Haushalte
persistent KontoHaushalte;

% Rückzahlungsdauer des Kredits
persistent Kreditrueckzahlungsdauer;

% Vermnögen der Bank aus den Gewinnen
persistent KontoBank;

% Summe Anzahl des Deckungsmaterials
persistent SummeDeckungsmaterial;

    % Zinsspread 1%
    if isempty(Zinsspread)
       Zinsspread = 0.01;
    end 
    
    % interner Zinssatz auf den Leitzins festlegen
    if isempty(InternerZinssatz)
       InternerZinssatz = 0.03;
    end     
    
    % Rückzahlungsdauer 15 Zeiteinheiten
    if isempty(Kreditrueckzahlungsdauer)
       Kreditrueckzahlungsdauer = 15;
    end     
   
    if isempty(KontoBank)
       KontoBank = 400;
    end   
    if isempty(KontoHaushalte)
       KontoHaushalte = 0;
    end   
    if isempty(KrediteHaushalte)
       KrediteHaushalte = 200;
    end     
    if isempty(KrediteUnternehmen)
       KrediteUnternehmen = 200;
    end 
    if isempty(KrediteStaat)
       KrediteStaat = 200;
    end     
    if isempty(KrediteUnternehmenAusland)
       KrediteUnternehmenAusland = 200;
    end     
    if isempty(KrediteHaushalteAusland)
       KrediteHaushalteAusland = 200;
    end   
    if isempty(SummeDeckungsmaterial)
       SummeDeckungsmaterial = 50;
    end       
    
    % Deckungsquote des Materials
    MindestDeckungsquote = 0.5;
    
    % Anfänglicher und maßgebliche Preis für das Deckungsmatrial
    InitPreisDeckungsmaterial = 10;   
        
    % Aufaddieren des Deckungsmaterials
    SummeDeckungsmaterial = SummeDeckungsmaterial + MengeDeckungsmaterial;
    
    % Habenzinsen berechnen
    HabenZinsen = KontoHaushalte * (InternerZinssatz - Zinsspread);
    KontoHaushalte = KontoHaushalte + HabenZinsen;
    
    % Ein- / Auszahlung
    KontoHaushalte = KontoHaushalte + EinlagenAenderungHaushalte;    
      
    % Maximale Kreditvergabe anhand der MindestDeckungsquote mit dem Deckungsmaterial
    % in Anhängigkeit von Preis
    MaximaleKreditvergabe = SummeDeckungsmaterial * InitPreisDeckungsmaterial * (1 / MindestDeckungsquote); 
   
    Gesamtkredit = KrediteHaushalte + KrediteUnternehmen + KrediteStaat;
    
    if Gesamtkredit > 20000
        Gesamtkredit= 20000;
    end
    
    MaximaleKreditvergabeUebrig = MaximaleKreditvergabe - Gesamtkredit;

    % Wenn genug Geld auf dem Konto ist, so wird ein prozenualer Anteil mit
    % dem neuen Kreditbedarf verrechnet ==> 10 %    
    if KontoHaushalte > KreditbedarfHaushalte && KreditbedarfHaushalte > 0
       AusgleichbarerGeldBedarf = KreditbedarfHaushalte * 0.1;
       KontoHaushalte = KontoHaushalte - AusgleichbarerGeldBedarf;
       KreditbedarfHaushalte = KreditbedarfHaushalte - AusgleichbarerGeldBedarf;
    end         

    % Kreditberechnung für Haushalte      
    [KrediteHaushalte, KreditvergabeHaushalte, KreditrueckzahlungHaushalte, ...
                        SollZinsenHaushalte, MaximaleKreditvergabeUebrig] = ...
        Kreditberechnung(KrediteHaushalte, KreditbedarfHaushalte, MaximaleKreditvergabeUebrig, ...
                        InternerZinssatz, Zinsspread, Kreditrueckzahlungsdauer);                    
    
    % Kreditberechnung für Staat   
    [KrediteStaat, KreditvergabeStaat, KreditrueckzahlungStaat, SollZinsenStaat, ...
                        MaximaleKreditvergabeUebrig] = ...
        Kreditberechnung(KrediteStaat, KreditbedarfStaat, MaximaleKreditvergabeUebrig, ...
                        InternerZinssatz, Zinsspread, Kreditrueckzahlungsdauer);                    

    % Kreditberechnung für Unternehmen   
    [KrediteUnternehmen, KreditvergabeUnternehmen, KreditrueckzahlungUnternehmen, ...
                        SollZinsenUnternehmen, MaximaleKreditvergabeUebrig] = ...
        Kreditberechnung(KrediteUnternehmen, KreditbedarfUnternehmen, MaximaleKreditvergabeUebrig, ...
                        InternerZinssatz, Zinsspread, Kreditrueckzahlungsdauer);

    % Kreditberechnung für Haushalte im Ausland
    [KrediteHaushalteAusland, KreditvergabeHaushalteAusland, KreditrueckzahlungHaushalteAusland, ...
                        SollZinsenHaushalteAusland, MaximaleKreditvergabeUebrig] = ...
        Kreditberechnung(KrediteHaushalteAusland, KreditbedarfHaushalteAusland, MaximaleKreditvergabeUebrig, ...
                        InternerZinssatz, Zinsspread, Kreditrueckzahlungsdauer);                                        

    % Kreditberechnung für Unternehmen im Ausland
    [KrediteUnternehmenAusland, KreditvergabeUnternehmenAusland, KreditrueckzahlungUnternehmenAusland, ...
                        SollZinsenUnternehmenAusland, MaximaleKreditvergabeUebrig] = ...
        Kreditberechnung(KrediteUnternehmenAusland, KreditbedarfUnternehmenAusland, MaximaleKreditvergabeUebrig, ...
                        InternerZinssatz, Zinsspread, Kreditrueckzahlungsdauer);                    
                    
    
    % Bezahlen des Deckungsmaterials
    KontoBank = KontoBank - MengeDeckungsmaterial * PreisDeckungsmaterial;
                    
    % Gewinnberechnung der Bank
    SollZinsen = SollZinsenHaushalte + SollZinsenStaat + SollZinsenUnternehmen ...
                + SollZinsenHaushalteAusland + SollZinsenUnternehmenAusland;
    Bankgewinn = SollZinsen - HabenZinsen - MengeDeckungsmaterial * PreisDeckungsmaterial; 
    
    % Steuerberechnung der Bank
    BankenSteuern = max(Bankgewinn * Steuersatz, 0);
    BankgewinnNachSteuern = Bankgewinn - BankenSteuern;
    
    % Kontostand der Bank berechnen
    KontoBank = KontoBank + Bankgewinn - BankenSteuern;
    
    % wenn nicht mehr viel Kredit vergeben werden kann, wird die Menge des
    % Deckungsmaterials aufgestockt
    if MaximaleKreditvergabeUebrig < Gesamtkredit * 0.1 && KontoBank >  (MengeDeckungsmaterial * PreisDeckungsmaterial * 1.1)
        NachfrageDeckungsmaterial = MengeDeckungsmaterial * 1.1 + 10;
    elseif KontoBank < 0
        NachfrageDeckungsmaterial = MengeDeckungsmaterial * 0.8;
    else
        NachfrageDeckungsmaterial = MengeDeckungsmaterial * 0.9;
    end
    
    % Zinssätze anpassen (Zinsänderung anpassen y = -0.00005x + 0.0025;
    Zinsaenderung = -0.00005 * BankgewinnNachSteuern + 0.001;
    Zinsaenderung = max(-0.01, min(Zinsaenderung, 0.01));
    
    if KontoHaushalte > Gesamtkredit
        Zinsaenderung = Zinsaenderung - 0.01;
    end
    
    InternerZinssatz = InternerZinssatz + Zinsaenderung;
    
    KrediteStaatOut = KrediteStaat;
    KrediteUnternehmenOut = KrediteUnternehmen;
    KrediteHaushalteOut = KrediteHaushalte;
    KrediteUnternehmenAuslandOut = KrediteUnternehmenAusland;
    KrediteHaushalteAuslandOut = KrediteHaushalteAusland;    
    KontoHaushalteOut = KontoHaushalte;    
    BankKontostand = KontoBank;
    Bankenzinssatz = InternerZinssatz;

== matlab function Waehrungsmodelle/Währungssystem4/Öffentliche Dienstleistungen/MATLAB Function ==
  data: Finanzierung input; ArbeitsplaetzeDienstleistung output; Erwerbsfaehige input; Arbeitslohn input; Dienstleistungsqualitaet output
function [ArbeitsplaetzeDienstleistung, Dienstleistungsqualitaet] = OeffentlicheDienstleistungen(Finanzierung, Erwerbsfaehige, Arbeitslohn)
%# Submodul zur Berechnung das Öffentliche Dienstleistungsmodell

    persistent Arbeitsplaetze;

    % Anfangsarbeitsplätze
    if isempty(Arbeitsplaetze)
       Arbeitsplaetze = 20;
    end 

    % Da der Arbeitslohn ein Referenzlohn der privaten Unternehmen ist wird
    % dieser angepasst und um 20 % gesenkt
    LohnNiveauOeffentlicherDienst = 0.8;
    Arbeitslohn = Arbeitslohn * LohnNiveauOeffentlicherDienst;
    
    % Es können nicht mehr Arbeitsplätze wie Erwerbsfähige vorhanden sind
    % besetzt werden
    if Erwerbsfaehige < Arbeitsplaetze
        Arbeitsplaetze = Erwerbsfaehige;
    end

    % Existiert nicht genug Geld für die öffentlichen Dientleistungen
    % werden die Arbeitsplätze an die Finanzierung vom Staat angepasst.
    if (Finanzierung < Arbeitsplaetze * Arbeitslohn)
        Arbeitsplaetze = floor(Finanzierung / Arbeitslohn);        
    end          
       
    ArbeitsplaetzeDienstleistung = Arbeitsplaetze;
    
    % Berechnet Dienstleistungsqualitaet mit min:0.2 und max:1
    % indem die Arbeitsplätze der öffentlichen Dienstleistungen durch die
    % gesamten Erwerbstätigen geteilt werden und als Ausgleichfaktor mit drei
    % multipliziert wird. Somit ist es optimal wenn min. 1/3 aller
    % Erwerbsfähigen bei den öffentlichen Dienstleistungen arbeiten
    Dienstleistungsqualitaet = max(0.2, min(1, 3 * Arbeitsplaetze / Erwerbsfaehige));
